simulink model "simulation_pivot"  (R2020a)
settings: Solver=VariableStepAuto  StartTime=0.0  StopTime=60.0  RelTol=1e-3
settings Model: Creator=loloche  LastModifiedBy=loloche

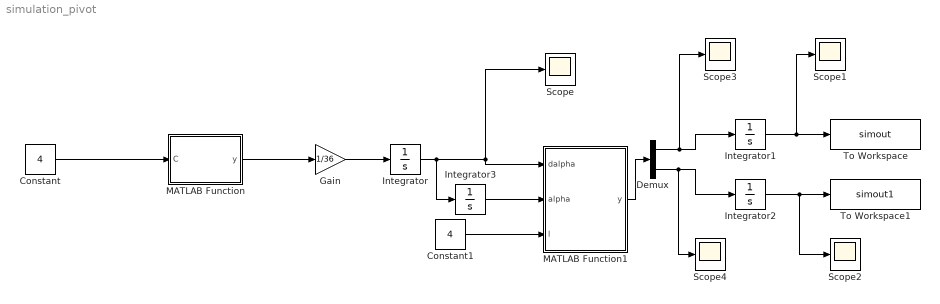
== system simulation_pivot ==
  Constant : Constant  Value=4
  Constant1 : Constant  Value=4
  Demux : Demux  Outputs=2
  Gain : Gain  Gain=1/36
  Integrator : Integrator
  Integrator1 : Integrator
  Integrator2 : Integrator  InitialCondition=2
  Integrator3 : Integrator
  MATLAB Function : MATLAB Function  TreatAsAtomicUnit=on
  MATLAB Function1 : MATLAB Function  TreatAsAtomicUnit=on
  Scope{,1..4} (5 alike) : Scope
  To Workspace : ToWorkspace  VariableName=simout  SaveFormat=Structure With Time  SampleTime=-1
  To Workspace1 : ToWorkspace  VariableName=simout1  SaveFormat=Structure With Time  SampleTime=-1
  wires:
  Constant/1 -> MATLAB Function/1(C)
  MATLAB Function/1(y) -> Gain/1
  Gain/1 -> Integrator/1
  Integrator/1 -> Integrator3/1, Scope/1, MATLAB Function1/1(dalpha)
  MATLAB Function1/1(y) -> Demux/1
  Demux/2 -> Scope4/1, Integrator2/1
  Demux/1 -> Scope3/1, Integrator1/1
  Integrator1/1 -> Scope1/1, To Workspace/1
  Integrator2/1 -> Scope2/1, To Workspace1/1
  Integrator3/1 -> MATLAB Function1/2(alpha)
  Constant1/1 -> MATLAB Function1/3(l)

== matlab function simulation_pivot/MATLAB Function1 ==
  data: dalpha input; y output; alpha input; l input
function y = fcn(dalpha, alpha, l)

y = [-dalpha*l*sin(alpha); dalpha*l*cos(alpha)];

== matlab function simulation_pivot/MATLAB Function ==
  data: C input; y output
function y = fcn(C)

y = C;
